simulink model "simulation_ACC_test"  (R2018b)
settings: Solver=ode2  StartTime=0.0  StopTime=90  FixedStep=0.4  RelTol=1e-3
undefined symbols (not defined in the file or in its folder): Delta_T, DiscIntNeverNeededParam, lead_bot_vel_vari, lead_bot_vel_vari_const, sigbuilder_block, timebpt
libraries: commchan3 x11, visionstatistics x4, simulink x3
(part 2 of 3)

== system simulation_ACC_test/Lead vehicle trajectory4 ==
  ego vehicle input : Inport
  Add1 : Sum  Inputs=-+
  Discrete-Time Integrator1 : DiscreteIntegrator  InitialCondition=0.6  SampleTime=-1  ICPrevOutput=DiscIntNeverNeededParam  ICPrevScaledInput=DiscIntNeverNeededParam
  Display : Display
  Display1 : Display
  Mux : Mux  Inputs=2
  Reshape : Reshape  OutputDimensionality=Column vector (2-D)
  Signal Builder : Subsystem  Tag=STV Subsys  LoadFcn=sigbuilder_block('load');  StartFcn=sigbuilder_block('start');  StopFcn=sigbuilder_block('stop');  ClipboardFcn=sigbuilder_block('clipboard');  mask(Sigbuilder block){tuvar=[0:10]}
      mask help: Simulink:masks:SigbuilderBlock_MD
      mask init:
      | if ~strcmp(get_param(bdroot(gcbh),'SimulationStatus'),'stopped') tuvar = sigbuilder_block('maskInit'); end
      settings: CopyFcn=sigbuilder_block('copy');  DeleteFcn=sigbuilder_block('delete');  ModelCloseFcn=sigbuilder_block('modelClose');  PreSaveFcn=sigbuilder_block('preSave');  PauseFcn=sigbuilder_block('pause');  ContinueFcn=sigbuilder_block('continue');  NameChangeFcn=sigbuilder_block('namechange');  OpenFcn=sigbuilder_block('open',[439.5 191.25 550.5 399.75 ]);  CloseFcn=sigbuilder_block('close');
      mask Display: plot(0, 0, 100, 100,[2, 2, 32, 32, 2], [68, 8, 8, 68, 68],[32, 2], [38, 38], [32, 19, 2],[53, 60, 44], [32, 17, 17, 2],[16, 16, 31, 31]);txt = getActiveGroup(gcbh);text(2, 100, txt,'verticalAlignment', 'top');
  Terminator : Terminator
  Terminator2 : Terminator
  Lead vehicle traject. and ego vehicle state out : Outport
  wires:
  Signal Builder/1(Position) -> Terminator/1
  Mux/1 -> Reshape/1
  Reshape/1 -> Display1/1, Add1/2
  Discrete-Time Integrator1/1 -> Mux/1
  ego vehicle input/1 -> Add1/1, Display/1
  Add1/1 -> Lead vehicle traject. and ego vehicle state out/1
  Signal Builder/3(Velocity const) -> Mux/2, Discrete-Time Integrator1/1
  Signal Builder/2(velocity step) -> Terminator2/1

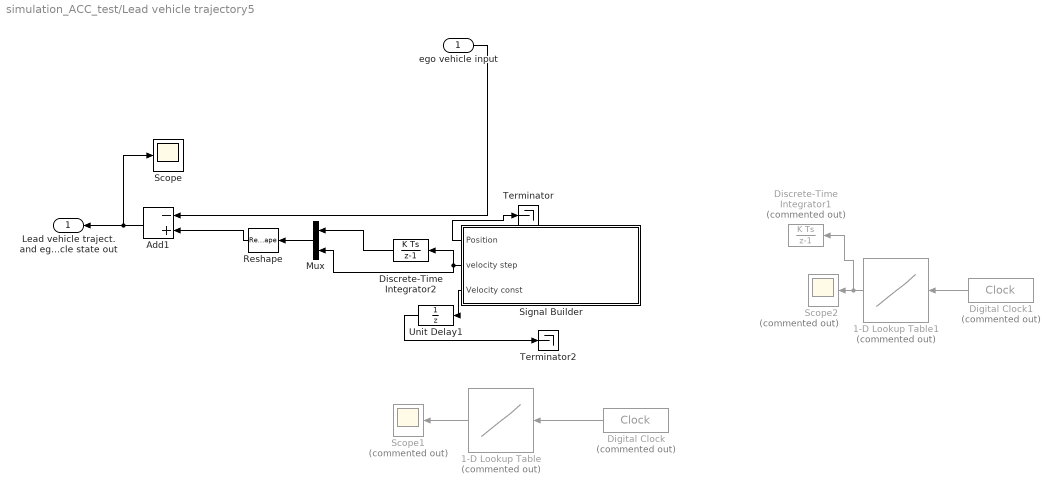
== system simulation_ACC_test/Lead vehicle trajectory5 ==
  ego vehicle input : Inport
  1-D Lookup Table : Lookup_n-D  Commented=on  NumberOfTableDimensions=1  BreakpointsForDimension1=timebpt  Table=lead_bot_vel_vari  ExtrapMethod=Clip  InternalRulePriority=Speed  RndMeth=Simplest  InputSameDT=on
  1-D Lookup Table1 : Lookup_n-D  Commented=on  NumberOfTableDimensions=1  BreakpointsForDimension1=timebpt  Table=lead_bot_vel_vari_const  ExtrapMethod=Clip  InternalRulePriority=Speed  RndMeth=Simplest  InputSameDT=on
  Add1 : Sum  Inputs=-+
  Digital Clock : DigitalClock  Commented=on  SampleTime=0.4
  Digital Clock1 : DigitalClock  Commented=on  SampleTime=0.4
  Discrete-Time Integrator1 : DiscreteIntegrator  Commented=on  SampleTime=-1  ICPrevOutput=DiscIntNeverNeededParam  ICPrevScaledInput=DiscIntNeverNeededParam
  Discrete-Time Integrator2 : DiscreteIntegrator  SampleTime=-1  ICPrevOutput=DiscIntNeverNeededParam  ICPrevScaledInput=DiscIntNeverNeededParam
  Mux : Mux  Inputs=2
  Reshape : Reshape  OutputDimensionality=Column vector (2-D)
  Scope : Scope
  Scope1 : Scope  Commented=on
  Scope2 : Scope  Commented=on
  Signal Builder : Subsystem  Tag=STV Subsys  LoadFcn=sigbuilder_block('load');  StartFcn=sigbuilder_block('start');  StopFcn=sigbuilder_block('stop');  ClipboardFcn=sigbuilder_block('clipboard');  mask(Sigbuilder block){tuvar=[0:10]}
      mask help: Simulink:masks:SigbuilderBlock_MD
      mask init:
      | if ~strcmp(get_param(bdroot(gcbh),'SimulationStatus'),'stopped') tuvar = sigbuilder_block('maskInit'); end
      settings: CopyFcn=sigbuilder_block('copy');  DeleteFcn=sigbuilder_block('delete');  ModelCloseFcn=sigbuilder_block('modelClose');  PreSaveFcn=sigbuilder_block('preSave');  PauseFcn=sigbuilder_block('pause');  ContinueFcn=sigbuilder_block('continue');  NameChangeFcn=sigbuilder_block('namechange');  OpenFcn=sigbuilder_block('open',[439.5 191.25 550.5 399.75 ]);  CloseFcn=sigbuilder_block('close');
      mask Display: plot(0, 0, 100, 100,[2, 2, 32, 32, 2], [68, 8, 8, 68, 68],[32, 2], [38, 38], [32, 19, 2],[53, 60, 44], [32, 17, 17, 2],[16, 16, 31, 31]);txt = getActiveGroup(gcbh);text(2, 100, txt,'verticalAlignment', 'top');
  Terminator : Terminator
  Terminator2 : Terminator
  Unit Delay1 : UnitDelay  SampleTime=-1
  Lead vehicle traject. and ego vehicle state out : Outport
  wires:
  Signal Builder/1(Position) -> Terminator/1
  Mux/1 -> Reshape/1
  Reshape/1 -> Add1/2
  ego vehicle input/1 -> Add1/1
  Add1/1 -> Scope/1, Lead vehicle traject. and ego vehicle state out/1
  Signal Builder/3(Velocity const) -> Unit Delay1/1
  Signal Builder/2(velocity step) -> Discrete-Time Integrator2/1, Mux/2
  Unit Delay1/1 -> Terminator2/1
  Digital Clock/1 -> 1-D Lookup Table/1
  1-D Lookup Table/1 -> Scope1/1
  1-D Lookup Table1/1 -> Discrete-Time Integrator1/1, Scope2/1
  Digital Clock1/1 -> 1-D Lookup Table1/1
  Discrete-Time Integrator2/1 -> Mux/1

== system simulation_ACC_test/New_1d_kalman_filter ==
  In1 : Inport
  A : Constant  Value=[1,0.4;0, 1]  VectorParams1D=off
  C : Constant  Value=[1, 0]  VectorParams1D=off
  MATLAB Function : MATLAB Function  TreatAsAtomicUnit=on
  Memory1 : Memory  InitialCondition=[0, 0]'  InheritSampleTime=on
  Process noise (Q) : Constant  Value=|  VectorParams1D=off
      | [0.0001, 0;
      | 0, 0.0001]
  Sensor noise variance (R) : Constant  Value=[0.0041]  VectorParams1D=off
  State estimation variance (P0) : Constant  Value=[0.0001, 0; 0, 0.0001]  VectorParams1D=off
  Out1 : Outport
  wires:
  MATLAB Function/1(sep) -> Out1/1
  Memory1/1 -> MATLAB Function/1("sem ")
  C/1 -> MATLAB Function/4(C)
  State estimation variance (P0)/1 -> MATLAB Function/7(P0)
  Sensor noise variance (R)/1 -> MATLAB Function/6(R)
  In1/1 -> MATLAB Function/2(sensor_data)
  Process noise (Q)/1 -> MATLAB Function/5(Q)
  A/1 -> MATLAB Function/3(A)
  MATLAB Function/2(sem) -> Memory1/1

== system simulation_ACC_test/New_1d_kalman_filter2 ==
  In1 : Inport
  A : Constant  Value=[1,0.4;0, 1]  VectorParams1D=off
  C : Constant  Value=[1, 0]  VectorParams1D=off
  MATLAB Function : MATLAB Function  TreatAsAtomicUnit=on
  Memory1 : Memory  InitialCondition=[0, 0]'  InheritSampleTime=on
  Process noise (Q) : Constant  Value=|  VectorParams1D=off
      | [0.0001, 0;
      | 0, 0.0001]
  Sensor noise variance (R) : Constant  Value=[0.0041]  VectorParams1D=off
  State estimation variance (P0) : Constant  Value=[0.0001, 0; 0, 0.0001]  VectorParams1D=off
  Out1 : Outport
  wires:
  MATLAB Function/1(sep) -> Out1/1
  Memory1/1 -> MATLAB Function/1("sem ")
  C/1 -> MATLAB Function/4(C)
  State estimation variance (P0)/1 -> MATLAB Function/7(P0)
  Sensor noise variance (R)/1 -> MATLAB Function/6(R)
  In1/1 -> MATLAB Function/2(sensor_data)
  Process noise (Q)/1 -> MATLAB Function/5(Q)
  A/1 -> MATLAB Function/3(A)
  MATLAB Function/2(sem) -> Memory1/1

== system simulation_ACC_test/Sensor Fusion ==
  simulated input : Inport
  2-D Mean : visionstatistics/2-D Mean  run=off  reset_popup=None  directionMode=Each row  dimension=1  treatSBRowAsCol=on  roiEnable=off  roiType=Rectangles  roiPortion=Entire ROI  roiOutput=Individual statistics for each ROI  roiFlag=off  outputDataTypeStr=Inherit: Same as accumulator  outputLastDataTypeStr=Inherit: Same as accumulator  outputMin=[]  outputMax=[]  accumMode=Binary point scaling  accumWordLength=32  accumFracLength=0  accumDataTypeStr=fixdt([],32,0)  accumLastDataTypeStr=fixdt([],32,0)  roundingMode=Floor  overflowMode=off
      settings: SourceProductName=Computer Vision System Toolbox  SourceProductBaseCode=VP
  Camera Sensor : Subsystem
  LDS sensor : Subsystem
  Matrix Concatenate : Concatenate  Mode=Multidimensional array  ConcatenateDimension=2
  New_1d_kalman_filter3 : Subsystem
  Scope6 : Scope
  lead vehicle speed : Outport
  Out2 : Outport  Port=2
  kalman out : Outport  Port=3
  sensor out : Outport  Port=4
  wires:
  2-D Mean/1 -> New_1d_kalman_filter3/1(In1), sensor out/1, Scope6/1
  simulated input/1 -> LDS sensor/1(Traject. input), Camera Sensor/1(Traject. input)
  Matrix Concatenate/1 -> 2-D Mean/1
  Camera Sensor/2(Sensor Output) -> Matrix Concatenate/2
  New_1d_kalman_filter3/1(Out1) -> kalman out/1
  LDS sensor/2(Sensor Output) -> Matrix Concatenate/1
  LDS sensor/1(Act lead vehicle speed) -> Out2/1
  Camera Sensor/1(Act lead vehicle speed) -> lead vehicle speed/1

== system simulation_ACC_test/combined sensor4 ==
  Traject. input : Inport
  AWGN Channel : commchan3/AWGN Channel  InputProcessing=Columns as channels (frame based)  seed=67  noiseMode="Signal to noise ratio  (SNR)"  EbNodB=100  EsNodB=10  SNRdB=11.1  bitsPerSym=1  Ps=1  Tsym=0.4  variance=1
  C : Constant  Commented=on  Value=[1, 0]  VectorParams1D=off
  Scope4 : Scope
  Scope7 : Scope
  sensor rel. distance : Outport
  Sensor Output : Outport  Port=2
  wires:
  Traject. input/1 -> sensor rel. distance/1, AWGN Channel/1, Scope7/1, Scope4/1  "Trajectory input"
  AWGN Channel/1 -> Sensor Output/1  "Sensor output"

== system simulation_ACC_test/Lead vehicle trajectory/Signal Builder ==
  Demux : Demux  Tag=STV Demux  Outputs=3
  FromWs : FromWorkspace  Tag=STV FromWs  VariableName=tuvar  SampleTime=0
      SigBuilderData=|
      | common.afterFinalStr = 'Extrapolate'
      | common.sampleTime = 0
      | dataSet.timeRange = [0 120]
      | dataSet.name = 'Group 1'
      | sbobj.Groups.Name = 'Group 1'
      | sbobj.Groups.Signals(1).Name = 'Position'
      | sbobj.Groups.Signals(1).XData = [0 6 10 120]
      | sbobj.Groups.Signals(1).YData = [0 0.705 1 1]
      | sbobj.Groups.Signals(2).Name = 'velocity step'
      | sbobj.Groups.Signals(2).XData = [0 60 60 120]
      | sbobj.Groups.Signals(2).YData = [0.1 0.1 0.2 0.2]
      | sbobj.Groups.Signals(3).Name = 'Velocity const'
      | sbobj.Groups.Signals(3).XData = [0 60 120]
      | sbobj.Groups.Signals(3).YData = [0.07 0.07 0.07]
      | sbobj.Groups.TimeRange = [0 120]
  Position : Outport  Tag=STV Outport
  velocity step : Outport  Tag=STV Outport  Port=2
  Velocity const : Outport  Tag=STV Outport  Port=3
  wires:
  FromWs/1 -> Demux/1
  Demux/1 -> Position/1
  Demux/2 -> velocity step/1
  Demux/3 -> Velocity const/1

== system simulation_ACC_test/Lead vehicle trajectory1/Signal Builder ==
  Demux : Demux  Tag=STV Demux  Outputs=3
  FromWs : FromWorkspace  Tag=STV FromWs  VariableName=tuvar  SampleTime=0
      SigBuilderData=|
      | common.afterFinalStr = 'Extrapolate'
      | common.sampleTime = 0
      | dataSet.timeRange = [0 120]
      | dataSet.name = 'Group 1'
      | sbobj.Groups.Name = 'Group 1'
      | sbobj.Groups.Signals(1).Name = 'Position'
      | sbobj.Groups.Signals(1).XData = [0 6 10 120]
      | sbobj.Groups.Signals(1).YData = [0.6 0.705 1 1]
      | sbobj.Groups.Signals(2).Name = 'velocity step'
      | sbobj.Groups.Signals(2).XData = [0 60 60 120]
      | sbobj.Groups.Signals(2).YData = [0.1 0.1 0.2 0.2]
      | sbobj.Groups.Signals(3).Name = 'Velocity const'
      | sbobj.Groups.Signals(3).XData = [0 60 120]
      | sbobj.Groups.Signals(3).YData = [0.07 0.07 0.07]
      | sbobj.Groups.TimeRange = [0 120]
  Position : Outport  Tag=STV Outport
  velocity step : Outport  Tag=STV Outport  Port=2
  Velocity const : Outport  Tag=STV Outport  Port=3
  wires:
  FromWs/1 -> Demux/1
  Demux/1 -> Position/1
  Demux/2 -> velocity step/1
  Demux/3 -> Velocity const/1

== system simulation_ACC_test/Lead vehicle trajectory2/Signal Builder ==
  Demux : Demux  Tag=STV Demux  Outputs=3
  FromWs : FromWorkspace  Tag=STV FromWs  VariableName=tuvar  SampleTime=0
      SigBuilderData=|
      | common.afterFinalStr = 'Extrapolate'
      | common.sampleTime = 0
      | dataSet.timeRange = [0 120]
      | dataSet.name = 'Group 1'
      | sbobj.Groups.Name = 'Group 1'
      | sbobj.Groups.Signals(1).Name = 'Position'
      | sbobj.Groups.Signals(1).XData = [0 6 10 120]
      | sbobj.Groups.Signals(1).YData = [0.6 0.705 1 1]
      | sbobj.Groups.Signals(2).Name = 'velocity step'
      | sbobj.Groups.Signals(2).XData = [0 60 60 120]
      | sbobj.Groups.Signals(2).YData = [0.1 0.1 0.2 0.2]
      | sbobj.Groups.Signals(3).Name = 'Velocity const'
      | sbobj.Groups.Signals(3).XData = [0 60 120]
      | sbobj.Groups.Signals(3).YData = [0.07 0.07 0.07]
      | sbobj.Groups.TimeRange = [0 120]
  Position : Outport  Tag=STV Outport
  velocity step : Outport  Tag=STV Outport  Port=2
  Velocity const : Outport  Tag=STV Outport  Port=3
  wires:
  FromWs/1 -> Demux/1
  Demux/1 -> Position/1
  Demux/2 -> velocity step/1
  Demux/3 -> Velocity const/1

== system simulation_ACC_test/Lead vehicle trajectory3/Signal Builder ==
  Demux : Demux  Tag=STV Demux  Outputs=3
  FromWs : FromWorkspace  Tag=STV FromWs  VariableName=tuvar  SampleTime=0
      SigBuilderData=|
      | common.afterFinalStr = 'Extrapolate'
      | common.sampleTime = 0
      | dataSet.timeRange = [0 120]
      | dataSet.name = 'Group 1'
      | sbobj.Groups.Name = 'Group 1'
      | sbobj.Groups.Signals(1).Name = 'Position'
      | sbobj.Groups.Signals(1).XData = [0 6 10 120]
      | sbobj.Groups.Signals(1).YData = [0 0.705 1 1]
      | sbobj.Groups.Signals(2).Name = 'velocity step'
      | sbobj.Groups.Signals(2).XData = [0 60 60 120]
      | sbobj.Groups.Signals(2).YData = [0.1 0.1 0.2 0.2]
      | sbobj.Groups.Signals(3).Name = 'Velocity const'
      | sbobj.Groups.Signals(3).XData = [0 60 120]
      | sbobj.Groups.Signals(3).YData = [0.07 0.07 0.07]
      | sbobj.Groups.TimeRange = [0 120]
  Position : Outport  Tag=STV Outport
  velocity step : Outport  Tag=STV Outport  Port=2
  Velocity const : Outport  Tag=STV Outport  Port=3
  wires:
  FromWs/1 -> Demux/1
  Demux/1 -> Position/1
  Demux/2 -> velocity step/1
  Demux/3 -> Velocity const/1

== system simulation_ACC_test/Lead vehicle trajectory4/Signal Builder ==
  Demux : Demux  Tag=STV Demux  Outputs=3
  FromWs : FromWorkspace  Tag=STV FromWs  VariableName=tuvar  SampleTime=0
      SigBuilderData=|
      | common.afterFinalStr = 'Extrapolate'
      | common.sampleTime = 0
      | dataSet.timeRange = [0 120]
      | dataSet.name = 'Group 1'
      | sbobj.Groups.Name = 'Group 1'
      | sbobj.Groups.Signals(1).Name = 'Position'
      | sbobj.Groups.Signals(1).XData = [0 6 10 120]
      | sbobj.Groups.Signals(1).YData = [0.6 0.705 1 1]
      | sbobj.Groups.Signals(2).Name = 'velocity step'
      | sbobj.Groups.Signals(2).XData = [0 60 60 120]
      | sbobj.Groups.Signals(2).YData = [0.1 0.1 0.2 0.2]
      | sbobj.Groups.Signals(3).Name = 'Velocity const'
      | sbobj.Groups.Signals(3).XData = [0 60 120]
      | sbobj.Groups.Signals(3).YData = [0.07 0.07 0.07]
      | sbobj.Groups.TimeRange = [0 120]
  Position : Outport  Tag=STV Outport
  velocity step : Outport  Tag=STV Outport  Port=2
  Velocity const : Outport  Tag=STV Outport  Port=3
  wires:
  FromWs/1 -> Demux/1
  Demux/1 -> Position/1
  Demux/2 -> velocity step/1
  Demux/3 -> Velocity const/1

== system simulation_ACC_test/Lead vehicle trajectory5/Signal Builder ==
  Demux : Demux  Tag=STV Demux  Outputs=3
  FromWs : FromWorkspace  Tag=STV FromWs  VariableName=tuvar  SampleTime=0
      SigBuilderData=|
      | common.afterFinalStr = 'Extrapolate'
      | common.sampleTime = 0
      | dataSet.timeRange = [0 120]
      | dataSet.name = 'Group 1'
      | sbobj.Groups.Name = 'Group 1'
      | sbobj.Groups.Signals(1).Name = 'Position'
      | sbobj.Groups.Signals(1).XData = [0 6 10 120]
      | sbobj.Groups.Signals(1).YData = [0 0.705 1 1]
      | sbobj.Groups.Signals(2).Name = 'velocity step'
      | sbobj.Groups.Signals(2).XData = [0 60 60 120]
      | sbobj.Groups.Signals(2).YData = [0.1 0.1 0.2 0.2]
      | sbobj.Groups.Signals(3).Name = 'Velocity const'
      | sbobj.Groups.Signals(3).XData = [0 60 120]
      | sbobj.Groups.Signals(3).YData = [0.07 0.07 0.07]
      | sbobj.Groups.TimeRange = [0 120]
  Position : Outport  Tag=STV Outport
  velocity step : Outport  Tag=STV Outport  Port=2
  Velocity const : Outport  Tag=STV Outport  Port=3
  wires:
  FromWs/1 -> Demux/1
  Demux/1 -> Position/1
  Demux/2 -> velocity step/1
  Demux/3 -> Velocity const/1

== system simulation_ACC_test/Sensor Fusion/Camera Sensor ==
  Traject. input : Inport
  AWGN Channel : commchan3/AWGN Channel  InputProcessing=Columns as channels (frame based)  seed=67  noiseMode="Signal to noise ratio  (SNR)"  EbNodB=100  EsNodB=10  SNRdB=19  bitsPerSym=1  Ps=1  Tsym=0.4  variance=1
  C : Constant  Value="[1, 0;    0, 1]"  VectorParams1D=off
  Product2 : Product  Multiplication=Matrix(*)
  Scope4 : Scope
  Scope7 : Scope
  Act lead vehicle speed : Outport
  Sensor Output : Outport  Port=2
  wires:
  Traject. input/1 -> Product2/2, Scope4/1  "Trajectory input"
  AWGN Channel/1 -> Sensor Output/1  "Sensor output"
  C/1 -> Product2/1
  Product2/1 -> Act lead vehicle speed/1, AWGN Channel/1, Scope7/1  "Actual Lead vehicle speed"

== system simulation_ACC_test/Sensor Fusion/LDS sensor ==
  Traject. input : Inport
  AWGN Channel : commchan3/AWGN Channel  InputProcessing=Columns as channels (frame based)  seed=67  noiseMode="Signal to noise ratio  (SNR)"  EbNodB=100  EsNodB=10  SNRdB=27  bitsPerSym=1  Ps=1  Tsym=0.4  variance=1
  C : Constant  Value="[1, 0;    0, 1]"  VectorParams1D=off
  Product2 : Product  Multiplication=Matrix(*)
  Scope4 : Scope
  Scope7 : Scope
  Act lead vehicle speed : Outport
  Sensor Output : Outport  Port=2
  wires:
  Product2/1 -> Act lead vehicle speed/1, AWGN Channel/1, Scope7/1  "Actual Lead vehicle speed"
  C/1 -> Product2/1
  Traject. input/1 -> Product2/2, Scope4/1  "Trajectory input"
  AWGN Channel/1 -> Sensor Output/1  "Sensor output"

== system simulation_ACC_test/Sensor Fusion/New_1d_kalman_filter3 ==
  In1 : Inport
  A : Constant  Value=[1,0.4;0, 1]  VectorParams1D=off
  C : Constant  Value=[1, 0]  VectorParams1D=off
  MATLAB Function : MATLAB Function  TreatAsAtomicUnit=on
  Memory1 : Memory  InitialCondition=[0, 0]'  InheritSampleTime=on
  Process noise (Q) : Constant  Value=|  VectorParams1D=off
      | [0.0001, 0;
      | 0, 0.0001]
  Sensor noise variance (R) : Constant  Value=[0.0041]  VectorParams1D=off
  State estimation variance (P0) : Constant  Value=[0.0001, 0; 0, 0.0001]  VectorParams1D=off
  Out1 : Outport
  wires:
  MATLAB Function/1(sep) -> Out1/1
  Memory1/1 -> MATLAB Function/1("sem ")
  C/1 -> MATLAB Function/4(C)
  State estimation variance (P0)/1 -> MATLAB Function/7(P0)
  Sensor noise variance (R)/1 -> MATLAB Function/6(R)
  In1/1 -> MATLAB Function/2(sensor_data)
  Process noise (Q)/1 -> MATLAB Function/5(Q)
  A/1 -> MATLAB Function/3(A)
  MATLAB Function/2(sem) -> Memory1/1

== matlab function simulation_ACC_test/MATLAB Function1 ==
  data: x input; x_next output
function x_next = fcn(x)
% format for input
% x= [x, y, vx, vy];
% u = [vx; vy];
dt = 0.4;
% A = [1, 0, dt, 0;
%      0, 1, 0, dt;
%      0, 0, 1, 0;
%      0, 0, 0, 1];
% x= [x; vx];
 A = [1, dt;
     0, 1];
 %B = [0, 0, 1, 1];
  x_next = reshape((A * x),2,1); %+ B*u;

== matlab function simulation_ACC_test/MATLAB Function5 ==
  data: x input; y output
function y = fcn(x)
%x = [x; y; vx; vy];
% persistent temp
% 
% if isempty(temp)
%     temp = [0.8;0.8];
%     flag = 1;
% else
%     flag = 0;
% end
C = [1, 0;
    0, 1];
% if flag == 1
%     y = C * temp;
% else
    y = reshape((C * x),2,1);
end

== matlab function simulation_ACC_test/MATLAB Function2 ==
  data: x input; x_next output
function x_next = fcn(x)
% format for input
% x= [x, y, vx, vy];
% u = [vx; vy];
dt = 0.4;
% A = [1, 0, dt, 0;
%      0, 1, 0, dt;
%      0, 0, 1, 0;
%      0, 0, 0, 1];
% x= [x; vx];
 A = [1, dt;
     0, 1];
 %B = [0, 0, 1, 1];
  x_next = reshape((A * x),2,1); %+ B*u;

== matlab function simulation_ACC_test/MATLAB Function3 ==
  data: x input; y output
function y = fcn(x)
%x = [x; y; vx; vy];
% persistent temp
% 
% if isempty(temp)
%     temp = [0.8;0.8];
%     flag = 1;
% else
%     flag = 0;
% end
C = [1, 0;
    0, 1];
% if flag == 1
%     y = C * temp;
% else
    y = reshape((C * x),2,1);
end

== matlab function simulation_ACC_test/MATLAB Function4 ==
  data: rel_velx input; accel_new output; rel_posx input; vel_egox input; stat output; x output
function [accel_new,stat, x] = acc_sim(rel_velx, rel_posx, vel_egox)

% ACC ago with MPC, solving QP problem: min (0.5*x'*H*x + f' * x) with
% linear inequality constraint A*x >= b
% speed: current speed
% accele_new: spit out acceleration to change the velocity of the turtlebot
% brake: stop while no movement of the lead vehicle vel_ego=0.
% rel_dist : rel_posx distance between the ego and lead vehicle.
% v_ego: cruise speed to maintain the minimum distance.
% max_dist: maximum relative distance to have ACC mode on, this is doing
% because to the sensors has some ranges such as lidar has 3.5 meter range
% and vision can also detect object till some distance. Therefore, in this
% case, the maximum distance should be 2.5 m to 3.0 m.
% vel_ego: to change the acceleration of the vehicle. this info will be
% taken from the imu of the vehicle/turtlebot.
% dist_safe: safe distance to be considered on the actual vehicle for braking but for
% this turtlebot application it is 0

% using reletive velocity minimization.
% Cost function to minimize J = |V - V_set|^2.
% Main constraint is Dis_rel - D_safe >= 0. which is derived through
% integral of velocity i .e. V * t >= D_safe.
%%%%%%%%%%%%%%%%%%%%%%%%%%%%%%%%%%%%%%%%%%%%%%%%%%%%%velocity model cost
%%%%%%%%%%%%%%%%%%%%%%%%%%%%%%%%%%%%%%%%%%%%%%%%%%%%%function
%{
persistent time_rel
currTime = datetime;

if isempty(time_rel)
    time_rel = currTime;
end
dt= seconds(currTime - time_rel);
%dt = 2;

D_safe = 0.30; % safe distance is 30 cm.
   
H = [2 -2; -2 2];
f = [0; 0];

% setting v_ego >=0 and v_set >=0, V * t >= D_safe, v_ego < 0.2, v_set < 0.2.
A = [ 0 dt; 1 0; 0 1];
b = [D_safe; 0; 0];

iA0 = true;
%iA0nxt = false(size(b)-[1, 0]);
iA0 = [iA0; false(size(b)-[1, 0])]; % iA0 = false(size(b));
Aeq = [0, 1]; % check with someone
beq = [double(rel_velx)]; % check with someone % change it to lead vehicle velocity

    
if dt==0
    accel_new = 0; % because of comparing afterwards.
else
    for iter = 1:10
        [L,p] = chol(H,'lower');
        Linv = inv(L);

        opt = mpcqpsolverOptions;

%cold start the solver, inequality constraints
        [x,stat, iA] = mpcqpsolver(Linv,f,A,b,Aeq,beq,iA0,opt);
        iA0 = iA;
   end

   if (stat > 0)
        accel_new = x(2,:);
    else
        accel_new = 0;
   end
end
%}
% persistent ini_ego_vel 
% if isempty(ini_ego_vel)
%     ini_ego_vel =0.01;
%     vel_egox = ini_ego_vel;
% end
%%% relative Distance cost function %%%%%%
% minimize J = |x_rel - x_des|^2
const_vel = 0.02; % to keep the velocity of the turtlebot.
x_des = 0.40; % minimum distance is 40 cm.
H = 2;
f= -2*x_des;
A = 1;
b = x_des;
iA0 = false(size(b));
Aeq = [];
beq = zeros(0,1);

[L,p] = chol(H,'lower');
Linv = inv(L);
Linv = reshape(Linv,1,1);

opt = mpcqpsolverOptions;

% PI constants
Kp = 0.7813; % checked and calculated through documentation: http://emanual.robotis.com/docs/en/dxl/x/xl430-w250/#velocity-i-gain
Ki = 0.0153; % checked and calculated through documentation: http://emanual.robotis.com/docs/en/dxl/x/xl430-w250/#velocity-i-gain

%cold start the solver, inequality constraints
[x,stat,iA] = mpcqpsolver(Linv,f,A,b,Aeq,beq,iA0,opt);
if rel_velx < 0
    rel_velx =0;
end

persistent err_old
if isempty(err_old)
    err_old = 0;
end

if rel_velx > -0.2 & rel_velx < 0.2
    if stat > 0
     %if x ~= x_des
        %accel_new = rel_velx + vel_egox + const_vel;
     %
        if rel_posx < x 
            accel_new = 0.0;
        else
           accel_new = ((rel_posx - x) * 0.4) + (rel_velx + vel_egox);% + const_vel;
            err = rel_posx - x;     % Positive error means vehicle is far.
            % err_old = err;
            int_err = err_old + ((err - err_old) * 0.4);
            accel_new = (Kp * err) + (Ki * int_err);
            err_old = err;           
        end
    else
        accel_new = vel_egox;
    end
else
    accel_new = vel_egox;
     %
    %{
    if rel_posx <= x & rel_posx >= 0.3
         accel_new = vel_egox; %0.0;
    elseif rel_posx <=0.25
        accel_new = 0.0;
    end
     %}
%  else
%      accel_new = 0.0;   
 end

% disp(['##1 -- Status : ',num2str(stat)])
% disp(['##2 -- relative position : ',num2str(rel_posx)])
% disp(['##2 -- ego velocity : ',num2str(vel_egox)])
% disp(['##2 -- relative velocity : ',num2str(rel_velx)])
% disp(['##2 -- Acceleration Command : ',num2str(accel_new)])
end

== matlab function simulation_ACC_test/1-D Kalman Filter/MATLAB Function5 ==
  data: A input; K output; C input; Q input; R input; Pm input
% This code has referred from
% https://www.cs.cmu.edu/~cga/dynopt/kalman/kalman.html and
% https://statweb.stanford.edu/~candes/acm116/Handouts/Kalman.pdf
% for more info check it out.
% as we are having longitudinal autonomy, therefore taking simple state transition matrix!!
function K  = sim_vel_est_kalman_filt_1D(A, C, Q, R, Pm)
%{
    C = [1, 0];
R = [0.000225];
Q = [0.0001, 0;
      0, 0.0001];
P0 = [0.0001, 0;
       0, 0.0001];
    
sem = [0, 0]';
          if detectionClusters{1, 1}.Measurement(1, :) >= 0.5
            Q = [(0.035 * detectionClusters{1, 1}.Measurement(1, :))^2, 0;
                    0,  (0.035 * detectionClusters{1, 1}.Measurement(1, :))^2];
          end
          if detectionClusters{1, 1}.Measurement(1, :) >= 0.5
                R = [(0.05*detectionClusters{1, 1}.Measurement(1, :))^2];
          end
          if detectionClusters{1, 1}.Measurement(1, :) >= 0.5
                P0 = [(0.035 * detectionClusters{1, 1}.Measurement(1, :))^2, 0;
                        0 , (0.035 * detectionClusters{1, 1}.Measurement(1, :))^2];
          end
          dt = toc(tStart);
          tStart = tic;
          A = [1, dt;
                0, 1];
%}
% designing the Kalman filter

for i = 1:1000
% measurement step

    S = C * Pm * C' + R;
    %K = Pm*C'*inv(S); % change this inverse thing to solve with solutions of linear equations.
    % changing to linear eq solution:
    K =  Pm*C' * inv(S); % as it is 1 D dividing it, but for matrix linsolve is the best to get the "K".

    Pp = Pm - K*C*Pm;
 % prediction step
    Pm = A*Pp*A' + Q;
end

 
end

== matlab function simulation_ACC_test/MATLAB Function6 ==
  data: rel_velx input; accel_new output; rel_posx input; vel_egox input; stat output; x output
function [accel_new,stat, x] = acc_sim(rel_velx, rel_posx, vel_egox)

% ACC ago with MPC, solving QP problem: min (0.5*x'*H*x + f' * x) with
% linear inequality constraint A*x >= b
% speed: current speed
% accele_new: spit out acceleration to change the velocity of the turtlebot
% brake: stop while no movement of the lead vehicle vel_ego=0.
% rel_dist : rel_posx distance between the ego and lead vehicle.
% v_ego: cruise speed to maintain the minimum distance.
% max_dist: maximum relative distance to have ACC mode on, this is doing
% because to the sensors has some ranges such as lidar has 3.5 meter range
% and vision can also detect object till some distance. Therefore, in this
% case, the maximum distance should be 2.5 m to 3.0 m.
% vel_ego: to change the acceleration of the vehicle. this info will be
% taken from the imu of the vehicle/turtlebot.
% dist_safe: safe distance to be considered on the actual vehicle for braking but for
% this turtlebot application it is 0

% using reletive velocity minimization.
% Cost function to minimize J = |V - V_set|^2.
% Main constraint is Dis_rel - D_safe >= 0. which is derived through
% integral of velocity i .e. V * t >= D_safe.
%%%%%%%%%%%%%%%%%%%%%%%%%%%%%%%%%%%%%%%%%%%%%%%%%%%%%velocity model cost
%%%%%%%%%%%%%%%%%%%%%%%%%%%%%%%%%%%%%%%%%%%%%%%%%%%%%function
%{
persistent time_rel
currTime = datetime;

if isempty(time_rel)
    time_rel = currTime;
end
dt= seconds(currTime - time_rel);
%dt = 2;

D_safe = 0.30; % safe distance is 30 cm.
   
H = [2 -2; -2 2];
f = [0; 0];

% setting v_ego >=0 and v_set >=0, V * t >= D_safe, v_ego < 0.2, v_set < 0.2.
A = [ 0 dt; 1 0; 0 1];
b = [D_safe; 0; 0];

iA0 = true;
%iA0nxt = false(size(b)-[1, 0]);
iA0 = [iA0; false(size(b)-[1, 0])]; % iA0 = false(size(b));
Aeq = [0, 1]; % check with someone
beq = [double(rel_velx)]; % check with someone % change it to lead vehicle velocity

    
if dt==0
    accel_new = 0; % because of comparing afterwards.
else
    for iter = 1:10
        [L,p] = chol(H,'lower');
        Linv = inv(L);

        opt = mpcqpsolverOptions;

%cold start the solver, inequality constraints
        [x,stat, iA] = mpcqpsolver(Linv,f,A,b,Aeq,beq,iA0,opt);
        iA0 = iA;
   end

   if (stat > 0)
        accel_new = x(2,:);
    else
        accel_new = 0;
   end
end
%}
% persistent ini_ego_vel 
% if isempty(ini_ego_vel)
%     ini_ego_vel =0.01;
%     vel_egox = ini_ego_vel;
% end
%%% relative Distance cost function %%%%%%
% minimize J = |x_rel - x_des|^2
const_vel = 0.02; % to keep the velocity of the turtlebot.
x_des = 0.40; % minimum distance is 40 cm.
H = 2;
f= -2*x_des;
A = 1;
b = x_des;
iA0 = false(size(b));
Aeq = [];
beq = zeros(0,1);

[L,p] = chol(H,'lower');
Linv = inv(L);
Linv = reshape(Linv,1,1);

opt = mpcqpsolverOptions;

% PI constants
Kp = 0.7813; % checked and calculated through documentation: http://emanual.robotis.com/docs/en/dxl/x/xl430-w250/#velocity-i-gain
Ki = 0.0153; % checked and calculated through documentation: http://emanual.robotis.com/docs/en/dxl/x/xl430-w250/#velocity-i-gain

%cold start the solver, inequality constraints
[x,stat,iA] = mpcqpsolver(Linv,f,A,b,Aeq,beq,iA0,opt);
if rel_velx < 0
    rel_velx =0;
end

persistent err_old
if isempty(err_old)
    err_old = 0;
end

if rel_velx > -0.2 & rel_velx < 0.2
    if stat > 0
     %if x ~= x_des
        %accel_new = rel_velx + vel_egox + const_vel;
     %
        if rel_posx < x 
            accel_new = 0.0;
        else
           accel_new = ((rel_posx - x) * 0.4) + (rel_velx + vel_egox);% + const_vel;
            err = rel_posx - x;     % Positive error means vehicle is far.
            % err_old = err;
            int_err = err_old + ((err - err_old) * 0.4);
            accel_new = (Kp * err) + (Ki * int_err);
            err_old = err;           
        end
    else
        accel_new = vel_egox;
    end
else
    accel_new = vel_egox;
     %
    %{
    if rel_posx <= x & rel_posx >= 0.3
         accel_new = vel_egox; %0.0;
    elseif rel_posx <=0.25
        accel_new = 0.0;
    end
     %}
%  else
%      accel_new = 0.0;   
 end

% disp(['##1 -- Status : ',num2str(stat)])
% disp(['##2 -- relative position : ',num2str(rel_posx)])
% disp(['##2 -- ego velocity : ',num2str(vel_egox)])
% disp(['##2 -- relative velocity : ',num2str(rel_velx)])
% disp(['##2 -- Acceleration Command : ',num2str(accel_new)])
end

== matlab function simulation_ACC_test/1-D Kalman Filter1/MATLAB Function5 ==
  data: A input; K output; C input; Q input; R input; Pm input
% This code has referred from
% https://www.cs.cmu.edu/~cga/dynopt/kalman/kalman.html and
% https://statweb.stanford.edu/~candes/acm116/Handouts/Kalman.pdf
% for more info check it out.
% as we are having longitudinal autonomy, therefore taking simple state transition matrix!!
function K  = sim_vel_est_kalman_filt_1D(A, C, Q, R, Pm)
%{
    C = [1, 0];
R = [0.000225];
Q = [0.0001, 0;
      0, 0.0001];
P0 = [0.0001, 0;
       0, 0.0001];
    
sem = [0, 0]';
          if detectionClusters{1, 1}.Measurement(1, :) >= 0.5
            Q = [(0.035 * detectionClusters{1, 1}.Measurement(1, :))^2, 0;
                    0,  (0.035 * detectionClusters{1, 1}.Measurement(1, :))^2];
          end
          if detectionClusters{1, 1}.Measurement(1, :) >= 0.5
                R = [(0.05*detectionClusters{1, 1}.Measurement(1, :))^2];
          end
          if detectionClusters{1, 1}.Measurement(1, :) >= 0.5
                P0 = [(0.035 * detectionClusters{1, 1}.Measurement(1, :))^2, 0;
                        0 , (0.035 * detectionClusters{1, 1}.Measurement(1, :))^2];
          end
          dt = toc(tStart);
          tStart = tic;
          A = [1, dt;
                0, 1];
%}
% designing the Kalman filter

for i = 1:1000
% measurement step

    S = C * Pm * C' + R;
    %K = Pm*C'*inv(S); % change this inverse thing to solve with solutions of linear equations.
    % changing to linear eq solution:
    K =  Pm*C' * inv(S); % as it is 1 D dividing it, but for matrix linsolve is the best to get the "K".

    Pp = Pm - K*C*Pm;
 % prediction step
    Pm = A*Pp*A' + Q;
end

 
end

== matlab function simulation_ACC_test/MATLAB Function7 ==
  data: rel_velx input; accel_new output; rel_posx input; vel_egox input; stat output; x output
function [accel_new,stat, x] = acc_sim(rel_velx, rel_posx, vel_egox)

% ACC ago with MPC, solving QP problem: min (0.5*x'*H*x + f' * x) with
% linear inequality constraint A*x >= b
% speed: current speed
% accele_new: spit out acceleration to change the velocity of the turtlebot
% brake: stop while no movement of the lead vehicle vel_ego=0.
% rel_dist : rel_posx distance between the ego and lead vehicle.
% v_ego: cruise speed to maintain the minimum distance.
% max_dist: maximum relative distance to have ACC mode on, this is doing
% because to the sensors has some ranges such as lidar has 3.5 meter range
% and vision can also detect object till some distance. Therefore, in this
% case, the maximum distance should be 2.5 m to 3.0 m.
% vel_ego: to change the acceleration of the vehicle. this info will be
% taken from the imu of the vehicle/turtlebot.
% dist_safe: safe distance to be considered on the actual vehicle for braking but for
% this turtlebot application it is 0

% using reletive velocity minimization.
% Cost function to minimize J = |V - V_set|^2.
% Main constraint is Dis_rel - D_safe >= 0. which is derived through
% integral of velocity i .e. V * t >= D_safe.
%%%%%%%%%%%%%%%%%%%%%%%%%%%%%%%%%%%%%%%%%%%%%%%%%%%%%velocity model cost
%%%%%%%%%%%%%%%%%%%%%%%%%%%%%%%%%%%%%%%%%%%%%%%%%%%%%function
%{
persistent time_rel
currTime = datetime;

if isempty(time_rel)
    time_rel = currTime;
end
dt= seconds(currTime - time_rel);
%dt = 2;

D_safe = 0.30; % safe distance is 30 cm.
   
H = [2 -2; -2 2];
f = [0; 0];

% setting v_ego >=0 and v_set >=0, V * t >= D_safe, v_ego < 0.2, v_set < 0.2.
A = [ 0 dt; 1 0; 0 1];
b = [D_safe; 0; 0];

iA0 = true;
%iA0nxt = false(size(b)-[1, 0]);
iA0 = [iA0; false(size(b)-[1, 0])]; % iA0 = false(size(b));
Aeq = [0, 1]; % check with someone
beq = [double(rel_velx)]; % check with someone % change it to lead vehicle velocity

    
if dt==0
    accel_new = 0; % because of comparing afterwards.
else
    for iter = 1:10
        [L,p] = chol(H,'lower');
        Linv = inv(L);

        opt = mpcqpsolverOptions;

%cold start the solver, inequality constraints
        [x,stat, iA] = mpcqpsolver(Linv,f,A,b,Aeq,beq,iA0,opt);
        iA0 = iA;
   end

   if (stat > 0)
        accel_new = x(2,:);
    else
        accel_new = 0;
   end
end
%}
% persistent ini_ego_vel 
% if isempty(ini_ego_vel)
%     ini_ego_vel =0.01;
%     vel_egox = ini_ego_vel;
% end
%%% relative Distance cost function %%%%%%
% minimize J = |x_rel - x_des|^2
const_vel = 0.02; % to keep the velocity of the turtlebot.
x_des = 0.40; % minimum distance is 40 cm.
H = 2;
f= -2*x_des;
A = 1;
b = x_des;
iA0 = false(size(b));
Aeq = [];
beq = zeros(0,1);

[L,p] = chol(H,'lower');
Linv = inv(L);
Linv = reshape(Linv,1,1);

opt = mpcqpsolverOptions;

% PI constants
Kp = 0.7813; % checked and calculated through documentation: http://emanual.robotis.com/docs/en/dxl/x/xl430-w250/#velocity-i-gain
Ki = 0.0153; % checked and calculated through documentation: http://emanual.robotis.com/docs/en/dxl/x/xl430-w250/#velocity-i-gain

%cold start the solver, inequality constraints
[x,stat,iA] = mpcqpsolver(Linv,f,A,b,Aeq,beq,iA0,opt);
if rel_velx < 0
    rel_velx =0;
end

persistent err_old
if isempty(err_old)
    err_old = 0;
end

%if rel_velx > -0.2 & rel_velx < 0.2
    if stat > 0
     %if x ~= x_des
        %accel_new = rel_velx + vel_egox + const_vel;
     %
        if rel_posx < x 
            accel_new = 0.0;
        else
           accel_new = ((rel_posx - x) * 0.4) + (rel_velx + vel_egox);% + const_vel;
            err = rel_posx - x;     % Positive error means vehicle is far.
            % err_old = err;
            int_err = err_old + ((err - err_old) * 0.4);
            accel_new = (Kp * err) + (Ki * int_err);
            err_old = err;           
        end
    else
        accel_new = vel_egox;
    end
%else
    %accel_new = vel_egox;
     %
    %{
    if rel_posx <= x & rel_posx >= 0.3
         accel_new = vel_egox; %0.0;
    elseif rel_posx <=0.25
        accel_new = 0.0;
    end
     %}
%  else
%      accel_new = 0.0;   
 %end

% disp(['##1 -- Status : ',num2str(stat)])
% disp(['##2 -- relative position : ',num2str(rel_posx)])
% disp(['##2 -- ego velocity : ',num2str(vel_egox)])
% disp(['##2 -- relative velocity : ',num2str(rel_velx)])
% disp(['##2 -- Acceleration Command : ',num2str(accel_new)])
end

== matlab function simulation_ACC_test/1-D Kalman Filter2/MATLAB Function5 ==
  data: A input; K output; C input; Q input; R input; Pm input
% This code has referred from
% https://www.cs.cmu.edu/~cga/dynopt/kalman/kalman.html and
% https://statweb.stanford.edu/~candes/acm116/Handouts/Kalman.pdf
% for more info check it out.
% as we are having longitudinal autonomy, therefore taking simple state transition matrix!!
function K  = sim_vel_est_kalman_filt_1D(A, C, Q, R, Pm)
%{
    C = [1, 0];
R = [0.000225];
Q = [0.0001, 0;
      0, 0.0001];
P0 = [0.0001, 0;
       0, 0.0001];
    
sem = [0, 0]';
          if detectionClusters{1, 1}.Measurement(1, :) >= 0.5
            Q = [(0.035 * detectionClusters{1, 1}.Measurement(1, :))^2, 0;
                    0,  (0.035 * detectionClusters{1, 1}.Measurement(1, :))^2];
          end
          if detectionClusters{1, 1}.Measurement(1, :) >= 0.5
                R = [(0.05*detectionClusters{1, 1}.Measurement(1, :))^2];
          end
          if detectionClusters{1, 1}.Measurement(1, :) >= 0.5
                P0 = [(0.035 * detectionClusters{1, 1}.Measurement(1, :))^2, 0;
                        0 , (0.035 * detectionClusters{1, 1}.Measurement(1, :))^2];
          end
          dt = toc(tStart);
          tStart = tic;
          A = [1, dt;
                0, 1];
%}
% designing the Kalman filter

for i = 1:1000
% measurement step

    S = C * Pm * C' + R;
    %K = Pm*C'*inv(S); % change this inverse thing to solve with solutions of linear equations.
    % changing to linear eq solution:
    K =  Pm*C' * inv(S); % as it is 1 D dividing it, but for matrix linsolve is the best to get the "K".

    Pp = Pm - K*C*Pm;
 % prediction step
    Pm = A*Pp*A' + Q;
end

 
end

== matlab function simulation_ACC_test/MATLAB Function8 ==
  data: lead_velocity input; rel_velx input; accel_new output; rel_posx input; vel_egox input; stat output; x output
function [accel_new,stat, x] = acc_sim(lead_velocity, rel_velx, rel_posx, vel_egox)

% ACC ago with MPC, solving QP problem: min (0.5*x'*H*x + f' * x) with
% linear inequality constraint A*x >= b
% speed: current speed
% accele_new: spit out acceleration to change the velocity of the turtlebot
% brake: stop while no movement of the lead vehicle vel_ego=0.
% rel_dist : rel_posx distance between the ego and lead vehicle.
% v_ego: cruise speed to maintain the minimum distance.
% max_dist: maximum relative distance to have ACC mode on, this is doing
% because to the sensors has some ranges such as lidar has 3.5 meter range
% and vision can also detect object till some distance. Therefore, in this
% case, the maximum distance should be 2.5 m to 3.0 m.
% vel_ego: to change the acceleration of the vehicle. this info will be
% taken from the imu of the vehicle/turtlebot.
% dist_safe: safe distance to be considered on the actual vehicle for braking but for
% this turtlebot application it is 0

% using reletive velocity minimization.
% Cost function to minimize J = |V - V_set|^2.
% Main constraint is Dis_rel - D_safe >= 0. which is derived through
% integral of velocity i .e. V * t >= D_safe.
%%%%%%%%%%%%%%%%%%%%%%%%%%%%%%%%%%%%%%%%%%%%%%%%%%%%%velocity model cost
%%%%%%%%%%%%%%%%%%%%%%%%%%%%%%%%%%%%%%%%%%%%%%%%%%%%%function
%{
persistent time_rel
currTime = datetime;

if isempty(time_rel)
    time_rel = currTime;
end
dt= seconds(currTime - time_rel);
%dt = 2;

D_safe = 0.30; % safe distance is 30 cm.
   
H = [2 -2; -2 2];
f = [0; 0];

% setting v_ego >=0 and v_set >=0, V * t >= D_safe, v_ego < 0.2, v_set < 0.2.
A = [ 0 dt; 1 0; 0 1];
b = [D_safe; 0; 0];

iA0 = true;
%iA0nxt = false(size(b)-[1, 0]);
iA0 = [iA0; false(size(b)-[1, 0])]; % iA0 = false(size(b));
Aeq = [0, 1]; % check with someone
beq = [double(rel_velx)]; % check with someone % change it to lead vehicle velocity

    
if dt==0
    accel_new = 0; % because of comparing afterwards.
else
    for iter = 1:10
        [L,p] = chol(H,'lower');
        Linv = inv(L);

        opt = mpcqpsolverOptions;

%cold start the solver, inequality constraints
        [x,stat, iA] = mpcqpsolver(Linv,f,A,b,Aeq,beq,iA0,opt);
        iA0 = iA;
   end

   if (stat > 0)
        accel_new = x(2,:);
    else
        accel_new = 0;
   end
end
%}
% persistent ini_ego_vel 
% if isempty(ini_ego_vel)
%     ini_ego_vel =0.01;
%     vel_egox = ini_ego_vel;
% end
%%% relative Distance cost function %%%%%%
% minimize J = |x_rel - x_des|^2
const_vel = 0.02; % to keep the velocity of the turtlebot.
x_des = 0.40; % minimum distance is 40 cm.
H = 2;
f= -2*x_des;
A = 1;
b = x_des;
iA0 = false(size(b));
Aeq = [];
beq = zeros(0,1);

[L,p] = chol(H,'lower');
Linv = inv(L);
Linv = reshape(Linv,1,1);

opt = mpcqpsolverOptions;

% PI constants
Kp = 0.7813; % checked and calculated through documentation: http://emanual.robotis.com/docs/en/dxl/x/xl430-w250/#velocity-i-gain
Ki = 0.0153; % checked and calculated through documentation: http://emanual.robotis.com/docs/en/dxl/x/xl430-w250/#velocity-i-gain

%cold start the solver, inequality constraints
[x,stat,iA] = mpcqpsolver(Linv,f,A,b,Aeq,beq,iA0,opt);
if rel_velx < 0
    rel_velx =0;
end

% persistent err_old
% if isempty(err_old)
%     err_old = 0;
% end

%if rel_velx > -0.2 & rel_velx < 0.2
    if stat > 0
     %if x ~= x_des
        %accel_new = rel_velx + vel_egox + const_vel;
     %
        if rel_posx < x 
            accel_new = 0.0;
        else
           accel_new =  (rel_velx + vel_egox);
%             err = rel_posx - x;     % Positive error means vehicle is far.
%             % err_old = err;
%             int_err = err_old + ((err - err_old) * 0.4);
%             accel_new = (Kp * err) + (Ki * int_err);
%             err_old = err;           
        end
    else
           accel_new = 0;
    end
%else
    %accel_new = vel_egox;
     %
    %{
    if rel_posx <= x & rel_posx >= 0.3
         accel_new = vel_egox; %0.0;
    elseif rel_posx <=0.25
        accel_new = 0.0;
    end
     %}
%  else
%      accel_new = 0.0;   
 %end

% disp(['##1 -- Status : ',num2str(stat)])
% disp(['##2 -- relative position : ',num2str(rel_posx)])
% disp(['##2 -- ego velocity : ',num2str(vel_egox)])
% disp(['##2 -- relative velocity : ',num2str(rel_velx)])
% disp(['##2 -- Acceleration Command : ',num2str(accel_new)])
end

== matlab function simulation_ACC_test/MATLAB Function10 ==
  data: x input; x_next output
function x_next = fcn(x)
% format for input
% x= [x, y, vx, vy];
% u = [vx; vy];
dt = 0.4;
% A = [1, 0, dt, 0;
%      0, 1, 0, dt;
%      0, 0, 1, 0;
%      0, 0, 0, 1];
% x= [x; vx];
 A = [1, dt;
     0, 1];
 %B = [0, 0, 1, 1];
  x_next = reshape((A * x),2,1); %+ B*u;

== matlab function simulation_ACC_test/MATLAB Function11 ==
  data: x input; y output
function y = fcn(x)
%x = [x; y; vx; vy];
% persistent temp
% 
% if isempty(temp)
%     temp = [0.8;0.8];
%     flag = 1;
% else
%     flag = 0;
% end
C = [1, 0;
    0, 1];
% if flag == 1
%     y = C * temp;
% else
    y = reshape((C * x),2,1);
end

== matlab function simulation_ACC_test/MATLAB Function12 ==
  data: rel_velx input; accel_new output; rel_posx input; vel_egox input; stat output; x output
function [accel_new,stat, x] = acc_sim(rel_velx, rel_posx, vel_egox)

% ACC ago with MPC, solving QP problem: min (0.5*x'*H*x + f' * x) with
% linear inequality constraint A*x >= b
% speed: current speed
% accele_new: spit out acceleration to change the velocity of the turtlebot
% brake: stop while no movement of the lead vehicle vel_ego=0.
% rel_dist : rel_posx distance between the ego and lead vehicle.
% v_ego: cruise speed to maintain the minimum distance.
% max_dist: maximum relative distance to have ACC mode on, this is doing
% because to the sensors has some ranges such as lidar has 3.5 meter range
% and vision can also detect object till some distance. Therefore, in this
% case, the maximum distance should be 2.5 m to 3.0 m.
% vel_ego: to change the acceleration of the vehicle. this info will be
% taken from the imu of the vehicle/turtlebot.
% dist_safe: safe distance to be considered on the actual vehicle for braking but for
% this turtlebot application it is 0

% using reletive velocity minimization.
% Cost function to minimize J = |V - V_set|^2.
% Main constraint is Dis_rel - D_safe >= 0. which is derived through
% integral of velocity i .e. V * t >= D_safe.
%%%%%%%%%%%%%%%%%%%%%%%%%%%%%%%%%%%%%%%%%%%%%%%%%%%%%velocity model cost
%%%%%%%%%%%%%%%%%%%%%%%%%%%%%%%%%%%%%%%%%%%%%%%%%%%%%function
%{
persistent time_rel
currTime = datetime;

if isempty(time_rel)
    time_rel = currTime;
end
dt= seconds(currTime - time_rel);
%dt = 2;

D_safe = 0.30; % safe distance is 30 cm.
   
H = [2 -2; -2 2];
f = [0; 0];

% setting v_ego >=0 and v_set >=0, V * t >= D_safe, v_ego < 0.2, v_set < 0.2.
A = [ 0 dt; 1 0; 0 1];
b = [D_safe; 0; 0];

iA0 = true;
%iA0nxt = false(size(b)-[1, 0]);
iA0 = [iA0; false(size(b)-[1, 0])]; % iA0 = false(size(b));
Aeq = [0, 1]; % check with someone
beq = [double(rel_velx)]; % check with someone % change it to lead vehicle velocity

    
if dt==0
    accel_new = 0; % because of comparing afterwards.
else
    for iter = 1:10
        [L,p] = chol(H,'lower');
        Linv = inv(L);

        opt = mpcqpsolverOptions;

%cold start the solver, inequality constraints
        [x,stat, iA] = mpcqpsolver(Linv,f,A,b,Aeq,beq,iA0,opt);
        iA0 = iA;
   end

   if (stat > 0)
        accel_new = x(2,:);
    else
        accel_new = 0;
   end
end
%}
% persistent ini_ego_vel 
% if isempty(ini_ego_vel)
%     ini_ego_vel =0.01;
%     vel_egox = ini_ego_vel;
% end
%%% relative Distance cost function %%%%%%
% minimize J = |x_rel - x_des|^2
const_vel = 0.02; % to keep the velocity of the turtlebot.
x_des = 0.40; % minimum distance is 40 cm.
H = 2;
f= -2*x_des;
A = 1;
b = x_des;
iA0 = false(size(b));
Aeq = [];
beq = zeros(0,1);

[L,p] = chol(H,'lower');
Linv = inv(L);
Linv = reshape(Linv,1,1);

opt = mpcqpsolverOptions;

% PI constants
Kp = 0.7813; % checked and calculated through documentation: http://emanual.robotis.com/docs/en/dxl/x/xl430-w250/#velocity-i-gain
Ki = 0.0153; % checked and calculated through documentation: http://emanual.robotis.com/docs/en/dxl/x/xl430-w250/#velocity-i-gain

%cold start the solver, inequality constraints
[x,stat,iA] = mpcqpsolver(Linv,f,A,b,Aeq,beq,iA0,opt);
if rel_velx < 0
    rel_velx =0;
end

% persistent err_old
% if isempty(err_old)
%     err_old = 0;
% end

%if rel_velx > -0.2 & rel_velx < 0.2
    if stat > 0
     %if x ~= x_des
        %accel_new = rel_velx + vel_egox + const_vel;
     %
        if rel_posx < x 
            accel_new = 0.0;
        else
           accel_new =  (rel_velx + vel_egox);
%             err = rel_posx - x;     % Positive error means vehicle is far.
%             % err_old = err;
%             int_err = err_old + ((err - err_old) * 0.4);
%             accel_new = (Kp * err) + (Ki * int_err);
%             err_old = err;           
        end
    else
           accel_new = vel_egox;
    end
%else
    %accel_new = vel_egox;
     %
    %{
    if rel_posx <= x & rel_posx >= 0.3
         accel_new = vel_egox; %0.0;
    elseif rel_posx <=0.25
        accel_new = 0.0;
    end
     %}
%  else
%      accel_new = 0.0;   
 %end

% disp(['##1 -- Status : ',num2str(stat)])
% disp(['##2 -- relative position : ',num2str(rel_posx)])
% disp(['##2 -- ego velocity : ',num2str(vel_egox)])
% disp(['##2 -- relative velocity : ',num2str(rel_velx)])
% disp(['##2 -- Acceleration Command : ',num2str(accel_new)])
end

== matlab function simulation_ACC_test/MATLAB Function9 ==
  data: lead_velocity input; rel_velx input; accel_new output; rel_posx input; vel_egox input; stat output
function [accel_new, stat] = acc_sim(lead_velocity, rel_velx, rel_posx, vel_egox)

% ACC ago with MPC, solving QP problem: min (0.5*x'*H*x + f' * x) with
% linear inequality constraint A*x >= b
% speed: current speed
% accele_new: spit out acceleration to change the velocity of the turtlebot
% brake: stop while no movement of the lead vehicle vel_ego=0.
% rel_dist : rel_posx distance between the ego and lead vehicle.
% v_ego: cruise speed to maintain the minimum distance.
% max_dist: maximum relative distance to have ACC mode on, this is doing
% because to the sensors has some ranges such as lidar has 3.5 meter range
% and vision can also detect object till some distance. Therefore, in this
% case, the maximum distance should be 2.5 m to 3.0 m.
% vel_ego: to change the acceleration of the vehicle. this info will be
% taken from the imu of the vehicle/turtlebot.
% dist_safe: safe distance to be considered on the actual vehicle for braking but for
% this turtlebot application it is 0

% using reletive velocity minimization.
% Cost function to minimize J = |V - V_set|^2.
% Main constraint is Dis_rel - D_safe >= 0. which is derived through
% integral of velocity i .e. V * t >= D_safe.
%%%%%%%%%%%%%%%%%%%%%%%%%%%%%%%%%%%%%%%%%%%%%%%%%%%%%velocity model cost
%%%%%%%%%%%%%%%%%%%%%%%%%%%%%%%%%%%%%%%%%%%%%%%%%%%%%function
%{
persistent time_rel
currTime = datetime;

if isempty(time_rel)
    time_rel = currTime;
end
dt= seconds(currTime - time_rel);
%dt = 2;

D_safe = 0.30; % safe distance is 30 cm.
   
H = [2 -2; -2 2];
f = [0; 0];

% setting v_ego >=0 and v_set >=0, V * t >= D_safe, v_ego < 0.2, v_set < 0.2.
A = [ 0 dt; 1 0; 0 1];
b = [D_safe; 0; 0];

iA0 = true;
%iA0nxt = false(size(b)-[1, 0]);
iA0 = [iA0; false(size(b)-[1, 0])]; % iA0 = false(size(b));
Aeq = [0, 1]; % check with someone
beq = [double(rel_velx)]; % check with someone % change it to lead vehicle velocity

    
if dt==0
    accel_new = 0; % because of comparing afterwards.
else
    for iter = 1:10
        [L,p] = chol(H,'lower');
        Linv = inv(L);

        opt = mpcqpsolverOptions;

%cold start the solver, inequality constraints
        [x,stat, iA] = mpcqpsolver(Linv,f,A,b,Aeq,beq,iA0,opt);
        iA0 = iA;
   end

   if (stat > 0)
        accel_new = x(2,:);
    else
        accel_new = 0;
   end
end
%}
% persistent ini_ego_vel 
% if isempty(ini_ego_vel)
%     ini_ego_vel =0.01;
%     vel_egox = ini_ego_vel;
% end
%%% relative Distance cost function %%%%%%
% minimize J = |V - v_ego|^2
% const_vel = 0.02; % to keep the velocity of the turtlebot.
delta_t = 0.4;
x_des = 0.4; % minimum distance is 40 cm.
v_lead = rel_velx + vel_egox;
H = [2, 0; 
    0, 0.0001];
f= [-2*x_des; 0];
A = [0, 1;
    0, -1];
b = [0; -0.2];
iA0 = false(size(b));
Aeq = [1, delta_t];
beq = rel_posx + v_lead*delta_t;

[L,p] = chol(H,'lower');
Linv = inv(L);
%Linv = reshape(Linv,1,1);

opt = mpcqpsolverOptions;

% PI constants
Kp = 0.7813; % checked and calculated through documentation: http://emanual.robotis.com/docs/en/dxl/x/xl430-w250/#velocity-i-gain
Ki = 0.0153; % checked and calculated through documentation: http://emanual.robotis.com/docs/en/dxl/x/xl430-w250/#velocity-i-gain

%cold start the solver, inequality constraints
[x,stat,iA] = mpcqpsolver(Linv,f,A,b,Aeq,beq,iA0,opt);
if rel_velx < 0
    accel_new =0;
end

% persistent err_old
% if isempty(err_old)
%     err_old = 0;
% end

%if rel_velx > -0.2 & rel_velx < 0.2
    if stat > 0
     %if x ~= x_des
        %accel_new = rel_velx + vel_egox + const_vel;
     %
        accel_new =  x(2);
%             err = rel_posx - x;     % Positive error means vehicle is far.
%             % err_old = err;
%             int_err = err_old + ((err - err_old) * 0.4);
%             accel_new = (Kp * err) + (Ki * int_err);
%             err_old = err;           
    else
           accel_new = vel_egox;
    end
%else
    %accel_new = vel_egox;
     %
    %{
    if rel_posx <= x & rel_posx >= 0.3
         accel_new = vel_egox; %0.0;
    elseif rel_posx <=0.25
        accel_new = 0.0;
    end
     %}
%  else
%      accel_new = 0.0;   
 %end

% disp(['##1 -- Status : ',num2str(stat)])
% disp(['##2 -- relative position : ',num2str(rel_posx)])
% disp(['##2 -- ego velocity : ',num2str(vel_egox)])
% disp(['##2 -- relative velocity : ',num2str(rel_velx)])
% disp(['##2 -- Acceleration Command : ',num2str(accel_new)])
end
